simulink model "ship"  (Simulink 8.6)
settings: Solver=ode45  StartTime=0.0  StopTime=1000  RelTol=1e-3
values from neighbouring files (symbols this model uses):
  h_pd_d =     [matlab_1.mat]    (also in matlab_kalman_backup.mat)
  h_pd_n =     [matlab_1.mat]    (also in matlab_kalman_backup.mat)
  T_sample = 0.1    [DiscKal.m]    (also in kal_init.m)
libraries: simulink x2
settings Model: Creator=markh  LastModifiedBy=Magne
settings DataIOCC: SignalLoggingName=sigsOut
settings OptimizationCC: ExpressionDepthLimit=128  InitFltsAndDblsToZero=on
settings DebuggingCC: SaveWithParameterizedLinksMsg=none  SignalResolutionControl=TryResolveAllWithWarning  SolverPrmCheckMsg=none  MultiTaskDSMMsg=warning  MultiTaskCondExecSysMsg=none  FcnCallInpInsideContextMsg=UseLocalSettings
settings HardwareCC: TargetUnknown=on
settings GRTTargetCC: TargetFcnLib=ansi_tfl_tmw.mat

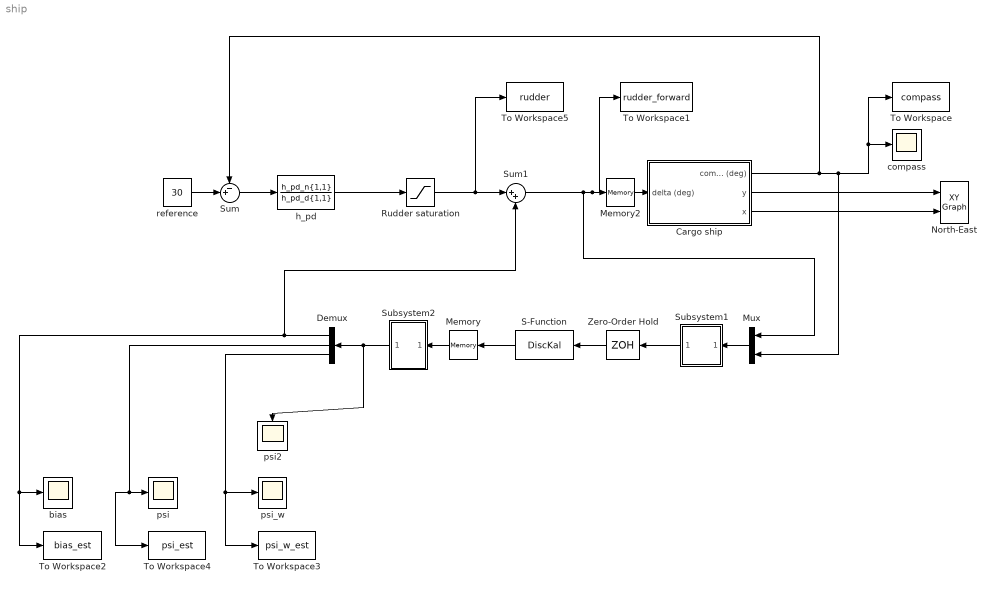
== system ship ==
  Cargo ship : Subsystem  mask(Simple shipmodel for a cargo ship){noise=on, current=on, logic=off}
      mask prompts: noise "measurement noise"; logic "waves"
      mask help:
      | Measurement noise:
      | 	checked = noise on
      | 	unchecked = noise off
      |
      | Current:
      | 	checked = current on
      | 	unchecked = current off
      |
      | Waves:
      | 	checked = waves on
      | 	unchecked = waves off
      |
      | Author: Jørgen Spjøtvold, 9/10-2003
      | TTK 4115 Linear system theory.
      | Modified by Jostein Bakkeheim 26/10-2006
  Demux : Demux  Outputs=3
  Memory : Memory
  Memory2 : Memory
  Mux : Mux  Inputs=2
  North-East : simulink/Sinks/XY Graph  xmin=-5000  xmax=5000  ymin=-5000  ymax=5000  st=-1
  Rudder saturation : Saturate  UpperLimit=45  LowerLimit=-45
  S-Function : S-Function  FunctionName=DiscKal  Parameters=data  SFunctionDeploymentMode=off  EnableBusSupport=off
  Subsystem1 : Subsystem  mask(degrees to radians){}
      mask help: Converts degrees to radians
      mask Display: fprintf('D2R');
  Subsystem2 : Subsystem  mask(radians to degrees){}
      mask help: Converts radians to degrees
      mask Display: fprintf('R2D');
  Sum : Sum  Inputs=-+|
  Sum1 : Sum  Inputs=|++
  To Workspace : ToWorkspace  VariableName=compass  SaveFormat=Timeseries  SampleTime=-1
  To Workspace1 : ToWorkspace  VariableName=rudder_forward  SaveFormat=Timeseries  SampleTime=-1
  To Workspace2 : ToWorkspace  VariableName=bias_est  SaveFormat=Timeseries  SampleTime=-1
  To Workspace3 : ToWorkspace  VariableName=psi_w_est  SaveFormat=Timeseries  SampleTime=-1
  To Workspace4 : ToWorkspace  VariableName=psi_est  SaveFormat=Timeseries  SampleTime=-1
  To Workspace5 : ToWorkspace  VariableName=rudder  SaveFormat=Timeseries  SampleTime=-1
  Zero-Order Hold : ZeroOrderHold  SampleTime=T_sample
  bias : Scope
  compass : Scope
  h_pd : TransferFcn  Numerator=h_pd_n{1,1}  Denominator=h_pd_d{1,1}
  psi : Scope
  psi2 : Scope
  psi_w : Scope
  reference : Constant  Value=30
  wires:
  Cargo ship/3(x) -> North-East/2
  Cargo ship/2(y) -> North-East/1
  Cargo ship/1(compass (deg)) -> Mux/2, To Workspace/1, compass/1, Sum/1
  Sum/1 -> h_pd/1
  reference/1 -> Sum/2
  Sum1/1 -> Mux/1, To Workspace1/1, Memory2/1
  Memory/1 -> Subsystem2/1(In1)
  Demux/1 -> Sum1/2, To Workspace2/1, bias/1
  Demux/2 -> To Workspace4/1, psi/1
  Demux/3 -> To Workspace3/1, psi_w/1
  S-Function/1 -> Memory/1
  Mux/1 -> Subsystem1/1(In1)
  Subsystem2/1(Out1) -> psi2/1, Demux/1
  Zero-Order Hold/1 -> S-Function/1
  Subsystem1/1(Out1) -> Zero-Order Hold/1
  Memory2/1 -> Cargo ship/1(delta (deg))
  h_pd/1 -> Rudder saturation/1
  Rudder saturation/1 -> To Workspace5/1, Sum1/1

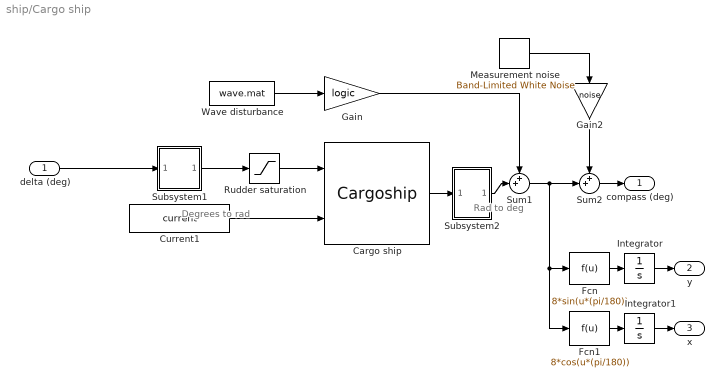
== system ship/Cargo ship ==
  note: Degrees to rad
  note: Rad to deg
  delta (deg) : Inport
  Cargo ship : S-Function  FunctionName=Cargoship  SFunctionDeploymentMode=off  EnableBusSupport=off  mask(Cargo ship){}
      mask help:
      | S-function which simulates a cargo ship.
      |
      | Author: Jørgen Spjøtvold
      | 20.10-2003
      | Modified by Jostein Bakkeheim 27.10.2006
  Current1 : Constant  Value=current
  Fcn : Fcn  Expr=8*sin(u*(pi/180))
  Fcn1 : Fcn  Expr=8*cos(u*(pi/180))
  Gain : Gain  Gain=logic  SaturateOnIntegerOverflow=on  OutDataTypeStr=Inherit: Same as input  ParamDataTypeStr=Inherit: Same as input
  Gain2 : Gain  Gain=noise  SaturateOnIntegerOverflow=on  OutDataTypeStr=Inherit: Same as input  ParamDataTypeStr=Inherit: Same as input
  Integrator : Integrator
  Integrator1 : Integrator
  Measurement noise : simulink/Sources/Band-Limited White Noise  Cov=[0.001]  Ts=.5  seed=[23341]
  Rudder saturation : Saturate  UpperLimit=45*(pi/180)  LowerLimit=-45*(pi/180)
  Subsystem1 : Subsystem  mask(degrees to radians){}
      mask help: Converts degrees to radians
      mask Display: fprintf('D2R');
  Subsystem2 : Subsystem  mask(radians to degrees){}
      mask help: Converts radians to degrees
      mask Display: fprintf('R2D');
  Sum1 : Sum  Inputs=++|  SaturateOnIntegerOverflow=on
  Sum2 : Sum  Inputs=++|  SaturateOnIntegerOverflow=on
  Wave disturbance : FromFile  FileName=wave.mat  SampleTime=0
  compass (deg) : Outport
  y : Outport  Port=2
  x : Outport  Port=3
  wires:
  delta (deg)/1 -> Subsystem1/1(In1)
  Fcn/1 -> Integrator/1
  Integrator/1 -> y/1
  Fcn1/1 -> Integrator1/1
  Integrator1/1 -> x/1
  Wave disturbance/1 -> Gain/1
  Subsystem2/1(Out1) -> Sum1/2
  Gain/1 -> Sum1/1
  Sum1/1 -> Fcn/1, Fcn1/1, Sum2/2
  Cargo ship/1 -> Subsystem2/1(In1)
  Subsystem1/1(Out1) -> Rudder saturation/1
  Rudder saturation/1 -> Cargo ship/1
  Sum2/1 -> compass (deg)/1
  Measurement noise/1 -> Gain2/1
  Gain2/1 -> Sum2/1
  Current1/1 -> Cargo ship/2

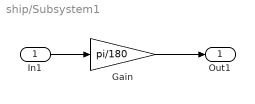
== system ship/Subsystem1 ==
  In1 : Inport
  Gain : Gain  Gain=pi/180  SaturateOnIntegerOverflow=on  OutDataTypeStr=Inherit: Same as input  ParamDataTypeStr=Inherit: Same as input
  Out1 : Outport
  wires:
  Gain/1 -> Out1/1
  In1/1 -> Gain/1

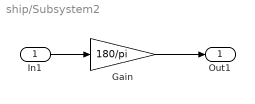
== system ship/Subsystem2 ==
  In1 : Inport
  Gain : Gain  Gain=180/pi  SaturateOnIntegerOverflow=on  OutDataTypeStr=Inherit: Same as input  ParamDataTypeStr=Inherit: Same as input
  Out1 : Outport
  wires:
  Gain/1 -> Out1/1
  In1/1 -> Gain/1

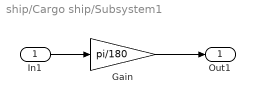
== system ship/Cargo ship/Subsystem1 ==
  In1 : Inport
  Gain : Gain  Gain=pi/180  SaturateOnIntegerOverflow=on  OutDataTypeStr=Inherit: Same as input  ParamDataTypeStr=Inherit: Same as input
  Out1 : Outport
  wires:
  Gain/1 -> Out1/1
  In1/1 -> Gain/1

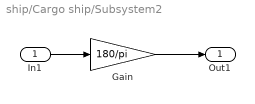
== system ship/Cargo ship/Subsystem2 ==
  In1 : Inport
  Gain : Gain  Gain=180/pi  SaturateOnIntegerOverflow=on  OutDataTypeStr=Inherit: Same as input  ParamDataTypeStr=Inherit: Same as input
  Out1 : Outport
  wires:
  Gain/1 -> Out1/1
  In1/1 -> Gain/1
